simulink model "second_order_smulink_model"  (R2024a)
settings: Solver=VariableStepAuto  StartTime=0.0  StopTime=1  RelTol=1e-3
settings Model: Creator=user  LastModifiedBy=user

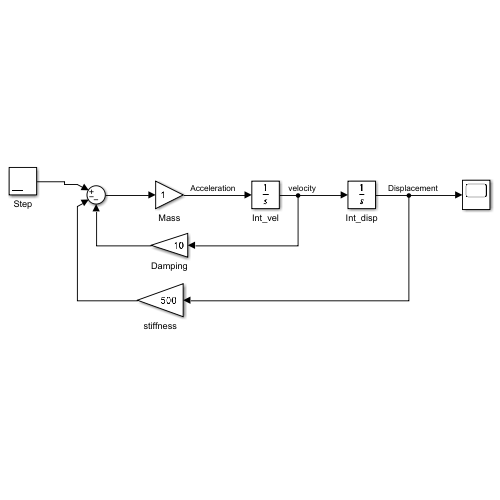
[thumbnail: Simulink's stored preview of the top-level diagram]
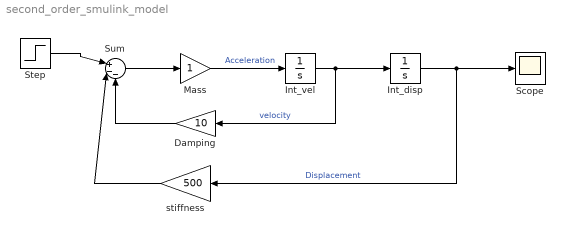
== system second_order_smulink_model ==
  Damping : Gain  Gain=10
  Int_disp : Integrator
  Int_vel : Integrator
  Mass : Gain
  Scope : Scope
  Step : Step  Time=0  SampleTime=0
  Sum : Sum  Inputs=|+--
  stiffness : Gain  Gain=500
  wires:
  Sum/1 -> Mass/1
  Mass/1 -> Int_vel/1  "Acceleration"
  Int_vel/1 -> Int_disp/1, Damping/1  "velocity"
  Int_disp/1 -> Scope/1, stiffness/1  "Displacement"
  Damping/1 -> Sum/3
  stiffness/1 -> Sum/2
  Step/1 -> Sum/1
